simulink model "FIRP_NL"  (R2021a)
settings: Solver=VariableStepAuto  StartTime=0.0  StopTime=10.0  RelTol=1e-3
values from neighbouring files (symbols this model uses):
  K = -(place(A,B,p))    [ass_7.m]
  L = Gamma - K*PI    [ass_7.m]
  w = 10    [ass_7.m]
settings Model: Creator=simon  LastModifiedBy=simon

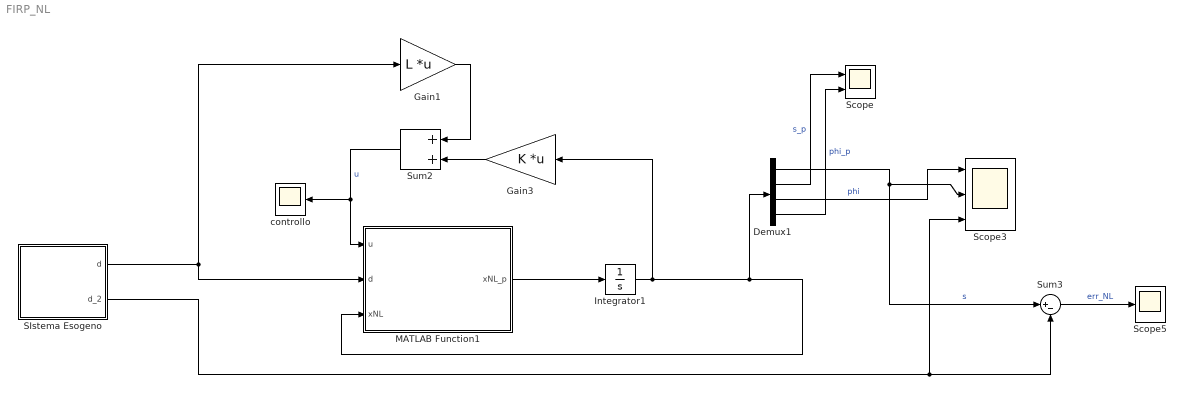
== system FIRP_NL ==
  Demux1 : Demux
  Gain1 : Gain  Gain=L  Multiplication=Matrix(K*u)
  Gain3 : Gain  Gain=K  Multiplication=Matrix(K*u)
  Integrator1 : Integrator
  MATLAB Function1 : MATLAB Function  TreatAsAtomicUnit=on
  SIstema Esogeno : Subsystem
  Scope : Scope  NumInputPorts=2
  Scope3 : Scope  NumInputPorts=3
  Scope5 : Scope
  Sum2 : Sum
  Sum3 : Sum  Inputs=|+-
  controllo : Scope
  wires:
  Sum3/1 -> Scope5/1  "err_NL"
  Gain3/1 -> Sum2/2
  MATLAB Function1/1(xNL_p) -> Integrator1/1
  Demux1/1 -> Sum3/1, Scope3/2  "s"
  Integrator1/1 -> Demux1/1, MATLAB Function1/3(xNL), Gain3/1
  Gain1/1 -> Sum2/1
  SIstema Esogeno/1(d) -> MATLAB Function1/2(d), Gain1/1
  SIstema Esogeno/2(d_2) -> Scope3/3, Sum3/2
  Sum2/1 -> controllo/1, MATLAB Function1/1(u)  "u"
  Demux1/3 -> Scope3/1  "phi"
  Demux1/2 -> Scope/1  "s_p"
  Demux1/4 -> Scope/2  "phi_p"

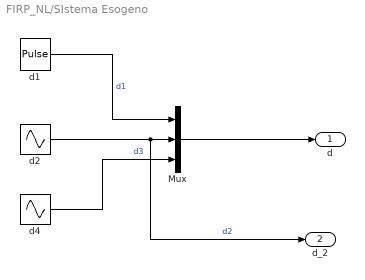
== system FIRP_NL/SIstema Esogeno ==
  Mux : Mux  Inputs=3
  d1 : DiscretePulseGenerator  PulseType=Time based  Amplitude=0.5  Period=50  PulseWidth=50
  d2 : Sin  Frequency=w  SampleTime=0
  d4 : Sin  Frequency=w  Phase=pi/2  SampleTime=0
  d : Outport
  d_2 : Outport  Port=2
  wires:
  d1/1 -> Mux/1  "d1"
  d2/1 -> d_2/1, Mux/2  "d2"
  d4/1 -> Mux/3  "d3"
  Mux/1 -> d/1

== matlab function FIRP_NL/MATLAB Function1 ==
  data: u input; xNL_p output; d input; xNL input
function xNL_p = NonLinearSpaceState(u,d,xNL)

M = 1;
l = 1;
F = 1;
g = 9.81;

xNL_p = zeros(4,1);

xNL_p(1)= xNL(2);
xNL_p(2)= (1/M)*(-F*xNL(2) + u + d(1));
xNL_p(3)= xNL(4);
xNL_p(4)= (g/l)*sin(xNL(3)) - (1/(M*l))*(-F*xNL(2) + u + d(1))*cos(xNL(3));
